simulink model "Thruster_Example_rw"  (R2024b)
settings: Solver=ode4  StartTime=0.0  StopTime=2000  FixedStep=0.01  RelTol=1e-3
undefined symbols (not defined in the file): Cube_L, dt, F_vec, Iws, M_rw, m_tot, norm_Ib, Omega1_init, Omega2_init, Omega3_init, Omega4_init, qb0, rad2rpm, RCS_F, RCS_F_vec, RCS_Pos, RCS_pos, RCS_PWM_Freq, RCS_Sampling_time, RCS_THR_vec, REL_TS_POS_I_0, REL_TS_VEL_I_0, RW_As, RW_Max_Speed, RW_Omegad_max, sat, SC_Ib, SC_state0, SS_Total_Mass, TC_Kepler, THR_dt, THR_Force, THR_freq, THR_Pos, TS_Ib, TS_qb0, TS_state0, TS_wb0, wb0, X, Y, Z
libraries: sm_lib x348, nesl_utility x236, simulink_extras x115, sharedtransform x64, aerolibutil x38, simulink x28, sharedutil x13
(part 8 of 16)

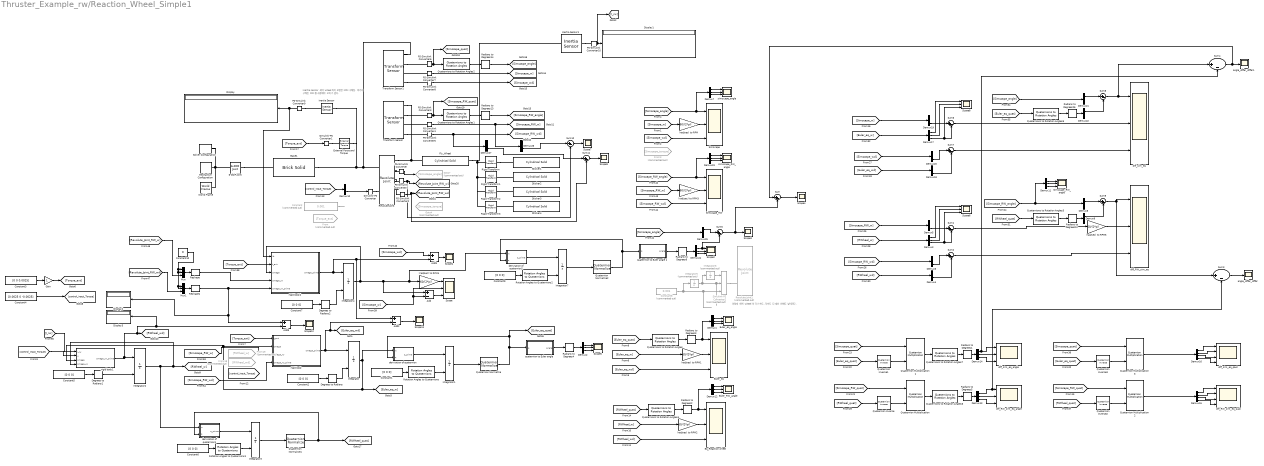
== system Thruster_Example_rw/Reaction_Wheel_Simple1 ==
  note: inertia sensor 써야 wheel까지 포함한 MOI 구해짐.
      | 여기서 구해진 MOI를 사용해야 오차가 없다.
  note: 이렇게 하면, wheel의 각가속도, 각속도 다 계산 안해도 넣어진다.
  (rad/sec) to RPM{,1..5} (6 alike) : Gain  Gain=60/(2*pi)
  6-DOF Joint : sm_lib/Joints/6-DOF Joint  JointMode=Normal  CompositeWrenchDir=FollowerOnBase  CompositeWrenchFrame=BaseFrame  SenseConstraintForce=off  SenseConstraintTorque=off  SenseTotalForce=off  SenseTotalTorque=off  PxPositionTargetSpecify=off  PxPositionTargetPriority=High  PxPositionTargetValue=0  PxPositionTargetValueUnits=m  PxVelocityTargetSpecify=off  PxVelocityTargetPriority=High  PxVelocityTargetValue=0  PxVelocityTargetValueUnits=m/s  PxEquilibriumPosition=0  PxEquilibriumPositionUnits=m  PxSpringStiffness=0  PxSpringStiffnessUnits=N/m  PxDampingCoefficient=0  PxDampingCoefficientUnits=N/(m/s)  PxLowerLimitSpecify=off  PxLowerLimitBound=-1  PxLowerLimitBoundUnits=m  PxLowerLimitStiffness=1e6  PxLowerLimitStiffnessUnits=N/m  PxLowerLimitDamping=1e3  PxLowerLimitDampingUnits=N/(m/s)  PxLowerLimitTransitionRegionWidth=1e-4  PxLowerLimitTransitionRegionWidthUnits=m  PxUpperLimitSpecify=off  PxUpperLimitBound=1  PxUpperLimitBoundUnits=m  PxUpperLimitStiffness=1e6  PxUpperLimitStiffnessUnits=N/m  PxUpperLimitDamping=1e3  PxUpperLimitDampingUnits=N/(m/s)  PxUpperLimitTransitionRegionWidth=1e-4  PxUpperLimitTransitionRegionWidthUnits=m  PxTorqueActuationMode=NoTorque  PxMotionActuationMode=ComputedMotion  PxSensePosition=off  PxSenseVelocity=off  PxSenseAcceleration=off  PxSenseTorqueForce=off  PxSenseLowerLimitTorqueForce=off  PxSenseUpperLimitTorqueForce=off  PyPositionTargetSpecify=off  PyPositionTargetPriority=High  PyPositionTargetValue=0  PyPositionTargetValueUnits=m  PyVelocityTargetSpecify=off  PyVelocityTargetPriority=High  PyVelocityTargetValue=0  PyVelocityTargetValueUnits=m/s  PyEquilibriumPosition=0  PyEquilibriumPositionUnits=m  PySpringStiffness=0  PySpringStiffnessUnits=N/m  PyDampingCoefficient=0  PyDampingCoefficientUnits=N/(m/s)  PyLowerLimitSpecify=off  PyLowerLimitBound=-1  PyLowerLimitBoundUnits=m  PyLowerLimitStiffness=1e6  PyLowerLimitStiffnessUnits=N/m  PyLowerLimitDamping=1e3  PyLowerLimitDampingUnits=N/(m/s)  PyLowerLimitTransitionRegionWidth=1e-4  PyLowerLimitTransitionRegionWidthUnits=m  PyUpperLimitSpecify=off  PyUpperLimitBound=1  PyUpperLimitBoundUnits=m  PyUpperLimitStiffness=1e6  PyUpperLimitStiffnessUnits=N/m  PyUpperLimitDamping=1e3  PyUpperLimitDampingUnits=N/(m/s)  PyUpperLimitTransitionRegionWidth=1e-4  PyUpperLimitTransitionRegionWidthUnits=m  PyTorqueActuationMode=NoTorque  PyMotionActuationMode=ComputedMotion  PySensePosition=off  PySenseVelocity=off  PySenseAcceleration=off  PySenseTorqueForce=off  PySenseLowerLimitTorqueForce=off  PySenseUpperLimitTorqueForce=off  PzPositionTargetSpecify=off  PzPositionTargetPriority=High  PzPositionTargetValue=0  PzPositionTargetValueUnits=m  PzVelocityTargetSpecify=off  PzVelocityTargetPriority=High  PzVelocityTargetValue=0  PzVelocityTargetValueUnits=m/s  PzEquilibriumPosition=0  PzEquilibriumPositionUnits=m  PzSpringStiffness=0  PzSpringStiffnessUnits=N/m  PzDampingCoefficient=0  PzDampingCoefficientUnits=N/(m/s)  PzLowerLimitSpecify=off  PzLowerLimitBound=-1  PzLowerLimitBoundUnits=m  PzLowerLimitStiffness=1e6  PzLowerLimitStiffnessUnits=N/m  PzLowerLimitDamping=1e3  PzLowerLimitDampingUnits=N/(m/s)  PzLowerLimitTransitionRegionWidth=1e-4  PzLowerLimitTransitionRegionWidthUnits=m  PzUpperLimitSpecify=off  PzUpperLimitBound=1  PzUpperLimitBoundUnits=m  PzUpperLimitStiffness=1e6  PzUpperLimitStiffnessUnits=N/m  PzUpperLimitDamping=1e3  PzUpperLimitDampingUnits=N/(m/s)  PzUpperLimitTransitionRegionWidth=1e-4  PzUpperLimitTransitionRegionWidthUnits=m  PzTorqueActuationMode=NoTorque  PzMotionActuationMode=ComputedMotion  PzSensePosition=off  PzSenseVelocity=off  PzSenseAcceleration=off  PzSenseTorqueForce=off  PzSenseLowerLimitTorqueForce=off  PzSenseUpperLimitTorqueForce=off  SphPositionTargetSpecify=off  SphPositionTargetPriority=High  SphPositionTargetRotationMethod=None  SphPositionTargetFollAlignAxisA=+X  SphPositionTargetBaseAlignAxisA=+Y  SphPositionTargetFollAlignAxisB=+Y  SphPositionTargetBaseAlignAxisB=+Z  SphPositionTargetRotationStandardAxis=+Z  SphPositionTargetRotationAngle=0.0  SphPositionTargetRotationAngleUnits=deg  SphPositionTargetRotationArbitraryAxis=[0 0 1]  SphPositionTargetRotationSequenceAxes=FollowerAxes  SphPositionTargetRotationSequence=XYX  SphPositionTargetRotationSequenceAngles=[0 0 0]  SphPositionTargetRotationSequenceAnglesUnits=deg  SphPositionTargetRotationMatrix=[1 0 0; 0 1 0; 0 0 1]  SphPositionTargetQuaternion=[1 0 0 0]  SphVelocityTargetSpecify=off  SphVelocityTargetPriority=High  SphVelocityTargetValue=[0 0 0]  SphVelocityTargetValueUnits=deg/s  SphVelocityTargetInFollowerFrame=on  SphEqPosRotationMethod=None  SphEqPosFollAlignAxisA=+X  SphEqPosBaseAlignAxisA=+Y  SphEqPosFollAlignAxisB=+Y  SphEqPosBaseAlignAxisB=+Z  SphEqPosRotationStandardAxis=+Z  SphEqPosRotationAngle=0.0  SphEqPosRotationAngleUnits=deg  SphEqPosRotationArbitraryAxis=[0 0 1]  SphEqPosRotationSequenceAxes=FollowerAxes  SphEqPosRotationSequence=XYX  SphEqPosRotationSequenceAngles=[0 0 0]  SphEqPosRotationSequenceAnglesUnits=deg  SphEqPosRotationMatrix=[1 0 0; 0 1 0; 0 0 1]  SphEqPosQuaternion=[1 0 0 0]  SphSpringStiffness=0  SphSpringStiffnessUnits=N*m/deg  SphDampingCoefficient=0  SphDampingCoefficientUnits=N*m/(deg/s)  SphLowerLimitSpecify=off  SphLowerLimitBound=15  SphLowerLimitBoundUnits=deg  SphLowerLimitStiffness=1e4  SphLowerLimitStiffnessUnits=N*m/deg  SphLowerLimitDamping=10  SphLowerLimitDampingUnits=N*m/(deg/s)  SphLowerLimitTransitionRegionWidth=0.1  SphLowerLimitTransitionRegionWidthUnits=deg  SphUpperLimitSpecify=off  SphUpperLimitBound=45  SphUpperLimitBoundUnits=deg  SphUpperLimitStiffness=1e4  SphUpperLimitStiffnessUnits=N*m/deg  SphUpperLimitDamping=10  SphUpperLimitDampingUnits=N*m/(deg/s)  SphUpperLimitTransitionRegionWidth=0.1  SphUpperLimitTransitionRegionWidthUnits=deg  SphTorqueActuationMode=NoTorque  SphActuateTorqueX=off  SphActuateTorqueY=off  SphActuateTorqueZ=on  SphActuateTorque=off  SphActuationFrame=BaseFrame  SphSensePosition=off  SphSenseVelocityX=off  SphSenseVelocityY=off  SphSenseVelocityZ=off  SphSenseVelocity=off  SphSenseAccelerationX=off  SphSenseAccelerationY=off  SphSenseAccelerationZ=off  SphSenseAcceleration=off  SphSenseLowerLimitTorqueMag=off  SphSenseUpperLimitTorqueMag=off  SphSensingFrame=BaseFrame
  Add{,1..3} (4 alike) : Sum  Inputs=+-
  Base1 : sm_lib/Body Elements/Brick Solid  BrickDimensions=[0.3 0.3 0.3]  BrickDimensionsUnits=m  ExportEntireGeometry=off  InertiaType=CalculateFromGeometry  BasedOnType=Mass  Density=1000  DensityUnits=kg/m^3  Mass=10  MassUnits=kg  CenterOfMass=[0 0 0]  CenterOfMassUnits=m  MomentsOfInertia=[1 1 1]  MomentsOfInertiaUnits=kg*m^2  ProductsOfInertia=[0 0 0]  ProductsOfInertiaUnits=kg*m^2  GraphicType=FromGeometry  MarkerShape=Sphere  MarkerSize=10  GraphicVisPropType=SimpleVisualProperties  GraphicDiffuseColor=[0.0 0.8 0.8]  GraphicOpacity=0.2  GraphicSpecularColor=[0.5 0.5 0.5 1.0]  GraphicAmbientColor=[0.15 0.15 0.15 1.0]  GraphicEmissiveColor=[0.0 0.0 0.0 1.0]  GraphicShininess=75  DoExposeReferenceFrame=on  SerializedFrames=<Frames><Frame><Id>Frame1</Id><Value><Name>CM_F</Name><Origin><Source>CenterOfMassFrame</Source><FeatureName></FeatureName></Origin><PrimaryAxis><DefinedDirection>+Z</DefinedDirection><Source>ReferenceFrame</Source><SourceDirection>+Z</SourceDirection><FeatureName></FeatureName></PrimaryAxis><SecondaryAxis><DefinedDirection>+X</DefinedDirection><Source>ReferenceFrame</Source><SourceDirection>+X</SourceDirection><FeatureName></FeatureName></SecondaryAxis></Value></Frame></Frames>
  Constant : Constant  Commented=on  Value=0.001
  Constant{1..2,5..7,9} (6 alike) : Constant  Value=[0 0 0]
  Constant10 : Constant  Value=0
  Constant3 : Constant  Value=[0 0 0.0025]
  Constant4 : Constant  Value=[0.0025 0 -0.0025]
  Constant8 : Constant  Commented=on  Value=0.001
  Degrees to Radians : simulink_extras/Transformations/Degrees to Radians
  Degrees to Radians1 : simulink_extras/Transformations/Degrees to Radians
  Degrees to Radians2 : simulink_extras/Transformations/Degrees to Radians
  Demux{1..14,17..27} (25 alike) : Demux  Outputs=3
  Demux15 : Demux
  Demux16 : Demux
  Display{,1..3} (4 alike) : Display
  Eq_Reaction wheel : Scope  NumInputPorts=3
  Euler_RW_angle : Scope  NumInputPorts=3
  Euler_eq : Scope  NumInputPorts=3
  Euler_eq_angle : Scope  NumInputPorts=3
  External Force and Torque : sm_lib/Forces and Torques/External Force and Torque  EnableForceX=off  EnableForceY=off  EnableForceZ=off  EnableForce=off  ForceResolutionFrame=World  EnableTorqueX=off  EnableTorqueY=off  EnableTorqueZ=off  EnableTorque=on  TorqueResolutionFrame=World
  Fly_Wheel : sm_lib/Body Elements/Cylindrical Solid  CylinderRadius=0.015  CylinderRadiusUnits=m  CylinderLength=0.01  CylinderLengthUnits=m  ExportEntireGeometry=off  InertiaType=CalculateFromGeometry  BasedOnType=Mass  Density=1000  DensityUnits=kg/m^3  Mass=0.01  MassUnits=kg  CenterOfMass=[0 0 0]  CenterOfMassUnits=m  MomentsOfInertia=[1 1 1]  MomentsOfInertiaUnits=kg*m^2  ProductsOfInertia=[0 0 0]  ProductsOfInertiaUnits=kg*m^2  GraphicType=FromGeometry  MarkerShape=Sphere  MarkerSize=10  GraphicVisPropType=SimpleVisualProperties  GraphicDiffuseColor=[0.0 0.0 1.0]  GraphicOpacity=1.0  GraphicSpecularColor=[0.5 0.5 0.5 1.0]  GraphicAmbientColor=[0.15 0.15 0.15 1.0]  GraphicEmissiveColor=[0.0 0.0 0.0 1.0]  GraphicShininess=75  DoExposeReferenceFrame=on  SerializedFrames=<Frames><Frame><Id>Frame1</Id><Value><Name>Sticker_F</Name><Origin><Source>GeometricFeature</Source><FeatureName>top surface</FeatureName></Origin><PrimaryAxis><DefinedDirection>+Z</DefinedDirection><Source>ReferenceFrame</Source><SourceDirection>+Z</SourceDirection><FeatureName></FeatureName></PrimaryAxis><SecondaryAxis><DefinedDirection>+X</DefinedDirection><Source>ReferenceFrame</Source><SourceDirection>+X</SourceDirection><FeatureName></FeatureName></SecondaryAxis></Value></Frame></Frames>
  From : From  Commented=on  GotoTag=Torque_ext
  From18 : From  Commented=on  GotoTag=RWheel_wd
  From19 : From  Commented=on  GotoTag=RWheel_w
  From3 : From  Commented=on  GotoTag=Simscape_torque
  Gain : Gain
  Goto4 : Goto  Commented=on  GotoTag=Simscape_torque
  Goto7 : Goto  Commented=on  GotoTag=Simscape_angle
  Inertia Sensor : sm_lib/Body Elements/Inertia Sensor  SensorExtent=Mechanism  SpanWeldJoints=off  ExcludeGroundedBodies=off  MeasurementFrame=Attached  SenseMass=off  SenseCenterOfMass=off  SenseInertiaMatrix=on  SenseCenteredInertiaMatrix=off  SensePrincipalInertiaMatrix=off  SenseRotationMatrix=off  GraphicType=PrincipalInertiaFrame  PrincipalInertiaFrameSize=20  GraphicVisPropType=SimpleVisualProperties  GraphicDiffuseColor=[0.5 0.5 0.5]  GraphicOpacity=1.0  GraphicSpecularColor=[0.5 0.5 0.5 1.0]  GraphicAmbientColor=[0.15 0.15 0.15 1.0]  GraphicEmissiveColor=[0.0 0.0 0.0 1.0]  GraphicShininess=75
  Inertia Sensor1 : sm_lib/Body Elements/Inertia Sensor  SensorExtent=BodyGroup  SpanWeldJoints=off  ExcludeGroundedBodies=off  MeasurementFrame=Attached  SenseMass=off  SenseCenterOfMass=off  SenseInertiaMatrix=on  SenseCenteredInertiaMatrix=off  SensePrincipalInertiaMatrix=off  SenseRotationMatrix=off  GraphicType=PrincipalInertiaFrame  PrincipalInertiaFrameSize=20  GraphicVisPropType=SimpleVisualProperties  GraphicDiffuseColor=[0.5 0.5 0.5]  GraphicOpacity=1.0  GraphicSpecularColor=[0.5 0.5 0.5 1.0]  GraphicAmbientColor=[0.15 0.15 0.15 1.0]  GraphicEmissiveColor=[0.0 0.0 0.0 1.0]  GraphicShininess=75
  Integrator{,1..4,7} (6 alike) : Integrator  InitialConditionSource=external
  Integrator5 : Integrator  Commented=on
  Integrator6 : Integrator  Commented=on
  Mechanism Configuration : sm_lib/Utilities/Mechanism Configuration  UniformGravity=None  GravityVector=[0 0 -9.80665]  GravityVectorUnits=m/s^2  LinearizationDelta=0.001  JointModeTransitionNonlinearIterations=2
  Mux : Mux  Inputs=3
  Mux1 : Mux  Inputs=3
  PS-Simulink Converter{,1..10} (11 alike) : nesl_utility/PS-Simulink Converter  PhysicalDomain=network_engine_domain  SubClassName=ps_output  LeftPortType=input  RightPortType=output  PseudoPeriodic=off  Frequencies=[]  VectorFormat=inherit  Unit=inherit  AffineConversion=off
  Quaternion Inverse{,1..3} (4 alike) : aerolibutil/Quaternion Inverse
  Quaternion Multiplication{,1..3} (4 alike) : aerolibutil/Quaternion Multiplication
  Quaternion Normalize : sharedutil/Quaternion Normalize  aMode=aMode
  Quaternion Normalize1 : sharedutil/Quaternion Normalize  aMode=aMode
  Quaternion Normalize2 : sharedutil/Quaternion Normalize  aMode=aMode
  Quaternions to Rotation Angles{,1..7} (8 alike) : sharedtransform/Quaternions to Rotation Angles  rotationOrder=ZYX  aMode=aMode
  Radians to Degrees{1..6,12..14,26} (10 alike) : simulink_extras/Transformations/Radians to Degrees
  Reshape : Reshape  OutputDimensionality=Column vector (2-D)
  Reshape1 : Reshape  OutputDimensionality=Column vector (2-D)
  Revolute Joint : sm_lib/Joints/Revolute Joint  JointMode=Normal  CompositeWrenchDir=FollowerOnBase  CompositeWrenchFrame=BaseFrame  SenseConstraintForce=off  SenseConstraintTorque=off  SenseTotalForce=off  SenseTotalTorque=off  PositionTargetSpecify=off  PositionTargetPriority=High  PositionTargetValue=0  PositionTargetValueUnits=deg  VelocityTargetSpecify=off  VelocityTargetPriority=High  VelocityTargetValue=0  VelocityTargetValueUnits=deg/s  EquilibriumPosition=0  EquilibriumPositionUnits=deg  SpringStiffness=0  SpringStiffnessUnits=N*m/deg  DampingCoefficient=0  DampingCoefficientUnits=N*m/(deg/s)  LowerLimitSpecify=off  LowerLimitBound=-90  LowerLimitBoundUnits=deg  LowerLimitStiffness=1e4  LowerLimitStiffnessUnits=N*m/deg  LowerLimitDamping=10  LowerLimitDampingUnits=N*m/(deg/s)  LowerLimitTransitionRegionWidth=0.1  LowerLimitTransitionRegionWidthUnits=deg  UpperLimitSpecify=off  UpperLimitBound=90  UpperLimitBoundUnits=deg  UpperLimitStiffness=1e4  UpperLimitStiffnessUnits=N*m/deg  UpperLimitDamping=10  UpperLimitDampingUnits=N*m/(deg/s)  UpperLimitTransitionRegionWidth=0.1  UpperLimitTransitionRegionWidthUnits=deg  TorqueActuationMode=InputTorque  MotionActuationMode=ComputedMotion  SensePosition=on  SenseVelocity=on  SenseAcceleration=on  SenseTorqueForce=on  SenseLowerLimitTorqueForce=off  SenseUpperLimitTorqueForce=off
  Revolute Joint1 : sm_lib/Joints/Revolute Joint  Commented=on  JointMode=Normal  CompositeWrenchDir=FollowerOnBase  CompositeWrenchFrame=BaseFrame  SenseConstraintForce=off  SenseConstraintTorque=off  SenseTotalForce=off  SenseTotalTorque=off  PositionTargetSpecify=off  PositionTargetPriority=High  PositionTargetValue=0  PositionTargetValueUnits=deg  VelocityTargetSpecify=off  VelocityTargetPriority=High  VelocityTargetValue=0  VelocityTargetValueUnits=deg/s  EquilibriumPosition=0  EquilibriumPositionUnits=deg  SpringStiffness=0  SpringStiffnessUnits=N*m/deg  DampingCoefficient=0  DampingCoefficientUnits=N*m/(deg/s)  LowerLimitSpecify=off  LowerLimitBound=-90  LowerLimitBoundUnits=deg  LowerLimitStiffness=1e4  LowerLimitStiffnessUnits=N*m/deg  LowerLimitDamping=10  LowerLimitDampingUnits=N*m/(deg/s)  LowerLimitTransitionRegionWidth=0.1  LowerLimitTransitionRegionWidthUnits=deg  UpperLimitSpecify=off  UpperLimitBound=90  UpperLimitBoundUnits=deg  UpperLimitStiffness=1e4  UpperLimitStiffnessUnits=N*m/deg  UpperLimitDamping=10  UpperLimitDampingUnits=N*m/(deg/s)  UpperLimitTransitionRegionWidth=0.1  UpperLimitTransitionRegionWidthUnits=deg  TorqueActuationMode=ComputedTorque  MotionActuationMode=InputMotion  SensePosition=on  SenseVelocity=on  SenseAcceleration=on  SenseTorqueForce=on  SenseLowerLimitTorqueForce=off  SenseUpperLimitTorqueForce=off
  Rigid Transform : sm_lib/Frames and Transforms/Rigid Transform  RotationMethod=None  FollAlignAxisA=+X  BaseAlignAxisA=+Y  FollAlignAxisB=+Y  BaseAlignAxisB=+Z  RotationStandardAxis=+Z  RotationAngle=0.0  RotationAngleUnits=deg  RotationArbitraryAxis=[0 0 1]  RotationSequenceAxes=FollowerAxes  RotationSequence=XYX  RotationSequenceAngles=[0 0 0]  RotationSequenceAnglesUnits=deg  RotationMatrix=[1 0 0; 0 1 0; 0 0 1]  Quaternion=[1 0 0 0]  TranslationMethod=Cartesian  TranslationCartesianOffset=[0.01 0 0]  TranslationCartesianOffsetUnits=m  TranslationStandardAxis=+Z  TranslationStandardOffset=0  TranslationStandardOffsetUnits=m  TranslationROffset=0  TranslationROffsetUnits=m  TranslationThetaOffset=0  TranslationThetaOffsetUnits=deg  TranslationZOffset=0  TranslationZOffsetUnits=m
  Rigid Transform1 : sm_lib/Frames and Transforms/Rigid Transform  RotationMethod=None  FollAlignAxisA=+X  BaseAlignAxisA=+Y  FollAlignAxisB=+Y  BaseAlignAxisB=+Z  RotationStandardAxis=+Z  RotationAngle=0.0  RotationAngleUnits=deg  RotationArbitraryAxis=[0 0 1]  RotationSequenceAxes=FollowerAxes  RotationSequence=XYX  RotationSequenceAngles=[0 0 0]  RotationSequenceAnglesUnits=deg  RotationMatrix=[1 0 0; 0 1 0; 0 0 1]  Quaternion=[1 0 0 0]  TranslationMethod=Cartesian  TranslationCartesianOffset=[-0.01 0 0]  TranslationCartesianOffsetUnits=m  TranslationStandardAxis=+Z  TranslationStandardOffset=0  TranslationStandardOffsetUnits=m  TranslationROffset=0  TranslationROffsetUnits=m  TranslationThetaOffset=0  TranslationThetaOffsetUnits=deg  TranslationZOffset=0  TranslationZOffsetUnits=m
  Rigid Transform2 : sm_lib/Frames and Transforms/Rigid Transform  RotationMethod=None  FollAlignAxisA=+X  BaseAlignAxisA=+Y  FollAlignAxisB=+Y  BaseAlignAxisB=+Z  RotationStandardAxis=+Z  RotationAngle=0.0  RotationAngleUnits=deg  RotationArbitraryAxis=[0 0 1]  RotationSequenceAxes=FollowerAxes  RotationSequence=XYX  RotationSequenceAngles=[0 0 0]  RotationSequenceAnglesUnits=deg  RotationMatrix=[1 0 0; 0 1 0; 0 0 1]  Quaternion=[1 0 0 0]  TranslationMethod=Cartesian  TranslationCartesianOffset=[0 0.01 0]  TranslationCartesianOffsetUnits=m  TranslationStandardAxis=+Z  TranslationStandardOffset=0  TranslationStandardOffsetUnits=m  TranslationROffset=0  TranslationROffsetUnits=m  TranslationThetaOffset=0  TranslationThetaOffsetUnits=deg  TranslationZOffset=0  TranslationZOffsetUnits=m
  Rigid Transform3 : sm_lib/Frames and Transforms/Rigid Transform  RotationMethod=None  FollAlignAxisA=+X  BaseAlignAxisA=+Y  FollAlignAxisB=+Y  BaseAlignAxisB=+Z  RotationStandardAxis=+Z  RotationAngle=0.0  RotationAngleUnits=deg  RotationArbitraryAxis=[0 0 1]  RotationSequenceAxes=FollowerAxes  RotationSequence=XYX  RotationSequenceAngles=[0 0 0]  RotationSequenceAnglesUnits=deg  RotationMatrix=[1 0 0; 0 1 0; 0 0 1]  Quaternion=[1 0 0 0]  TranslationMethod=Cartesian  TranslationCartesianOffset=[0 -0.01 0]  TranslationCartesianOffsetUnits=m  TranslationStandardAxis=+Z  TranslationStandardOffset=0  TranslationStandardOffsetUnits=m  TranslationROffset=0  TranslationROffsetUnits=m  TranslationThetaOffset=0  TranslationThetaOffsetUnits=deg  TranslationZOffset=0  TranslationZOffsetUnits=m
  Rotation Angles to Quaternions : sharedtransform/Rotation Angles to Quaternions  rotationOrder=ZYX  aMode=aMode
  Rotation Angles to Quaternions1 : sharedtransform/Rotation Angles to Quaternions  rotationOrder=ZYX  aMode=aMode
  Rotation Angles to Quaternions2 : sharedtransform/Rotation Angles to Quaternions  rotationOrder=ZYX  aMode=aMode
  Scope{,2,5..6,8} (5 alike) : Scope  NumInputPorts=3
  Scope{1,3..4,7,9,11..12} (7 alike) : Scope
  Simscape : Scope  NumInputPorts=3
  Simscape_RW : Scope  NumInputPorts=3
  Simscape_RW_angle : Scope  NumInputPorts=3
  Simulink-PS Converter : nesl_utility/Simulink-PS Converter  PhysicalDomain=network_engine_domain  SubClassName=ps_input  LeftPortType=input  RightPortType=output  PseudoPeriodic=off  Frequencies=[]  NoiseDistribution=none  NoiseParameters=[]  Unit=1  AffineConversion=off  FilteringAndDerivatives=provide  SimscapeFilterOrder=1  InputFilterTimeConstant=0.001  UdotUserProvided=0
  Simulink-PS Converter1 : nesl_utility/Simulink-PS Converter  PhysicalDomain=network_engine_domain  SubClassName=ps_input  LeftPortType=input  RightPortType=output  PseudoPeriodic=off  Frequencies=[]  NoiseDistribution=none  NoiseParameters=[]  Unit=1  AffineConversion=off  FilteringAndDerivatives=provide  SimscapeFilterOrder=1  InputFilterTimeConstant=0.001  UdotUserProvided=0
  Simulink-PS Converter2 : nesl_utility/Simulink-PS Converter  Commented=on  PhysicalDomain=network_engine_domain  SubClassName=ps_input  LeftPortType=input  RightPortType=output  PseudoPeriodic=off  Frequencies=[]  NoiseDistribution=none  NoiseParameters=[]  Unit=1  AffineConversion=off  FilteringAndDerivatives=provide  SimscapeFilterOrder=1  InputFilterTimeConstant=0.001  UdotUserProvided=2
  Solver Configuration : nesl_utility/Solver Configuration  PhysicalDomain=network_engine_domain  SubClassName=solver  LeftPortType=input  RightPortType=generic  Tones=[]  Harmonics=[]  SimulateNoise=off  Profile=off  UseLocalSampling=off  EnableSwitchedLinearOptims=on  FrequencyDomain=off  UseCCode=off  RelTol=0.001  AbsTol=0.001  MinStep=1e-09  ToWorkspace=off  RevertToSquareIcSolve=off  NumHomotopyIterations=100  PhasorMode=off  PhasorModeNumHarmonics=1  ConsistencySolver=NEWTON_XTOL_AFTER_FTOL  IndexReductionMethod=DerivativeReplacement  DoDC=off  ResidualTolerance=1e-09  ConsistencyTolSource=GLOBAL  ConsistencyAbsTol=0.001  ConsistencyRelTol=0.001  ConsistencyTolFactor=0.001  UseLocalSolver=off  LocalSolverChoice=NE_BACKWARD_EULER_ADVANCER  ResolveIndetEquations=on  FunctionEvalNumThread=1  LocalSolverSampleTime=0.001  DoFixedCost=off  MaxNonlinIter=3  MaxModeIter=2  ComputeImpulses=off  ImpulseIterations=2  LinearAlgebra=auto  LinearAlgebraNumThread=0  EquationFormulation=NE_TIME_EF  DelaysMemoryBudget=1024  AutomaticFiltering=on  FilteringTimeConstant=0.001  PartitionStorageMethod=AS_NEEDED  PartitionMemoryBudget=1024  PartitionMethod=ROBUST  MultibodyUseLocalSolver=off  MultibodyLocalSolverChoice=ODE1  MultibodyLocalSolverSampleTime=0.001
  Sticker{1..4} (4 alike) : sm_lib/Body Elements/Cylindrical Solid  CylinderRadius=0.003  CylinderRadiusUnits=m  CylinderLength=0.00001  CylinderLengthUnits=m  ExportEntireGeometry=off  InertiaType=CalculateFromGeometry  BasedOnType=Mass  Density=1000  DensityUnits=kg/m^3  Mass=0.000000000000000000000000000000000000000000000000000000000000000001  MassUnits=kg  CenterOfMass=[0 0 0]  CenterOfMassUnits=m  MomentsOfInertia=[1 1 1]  MomentsOfInertiaUnits=kg*m^2  ProductsOfInertia=[0 0 0]  ProductsOfInertiaUnits=kg*m^2  GraphicType=FromGeometry  MarkerShape=Sphere  MarkerSize=10  GraphicVisPropType=SimpleVisualProperties  GraphicDiffuseColor=[1.0 1.0 0.2]  GraphicOpacity=1.0  GraphicSpecularColor=[0.5 0.5 0.5 1.0]  GraphicAmbientColor=[0.15 0.15 0.15 1.0]  GraphicEmissiveColor=[0.0 0.0 0.0 1.0]  GraphicShininess=75  DoExposeReferenceFrame=on  SerializedFrames=<Frames><Frame><Id>Frame1</Id><Value><Name>Sticker_F</Name><Origin><Source>GeometricFeature</Source><FeatureName>bottom surface</FeatureName></Origin><PrimaryAxis><DefinedDirection>+Z</DefinedDirection><Source>ReferenceFrame</Source><SourceDirection>+Z</SourceDirection><FeatureName></FeatureName></PrimaryAxis><SecondaryAxis><DefinedDirection>+X</DefinedDirection><Source>ReferenceFrame</Source><SourceDirection>+X</SourceDirection><FeatureName></FeatureName></SecondaryAxis></Value></Frame></Frames>
  Sum{,1..11} (12 alike) : Sum  Inputs=|+-
  Transform Sensor : sm_lib/Frames and Transforms/Transform Sensor  MeasurementFrame=World  RotationSequence=ZYX  SenseAngle=off  SenseAxis=off  SenseQ=on  SenseR=off  SenseRotationSequence=off  SenseOmegaX=off  SenseOmegaY=off  SenseOmegaZ=off  SenseOmega=on  SenseQDot=off  SenseRDot=off  SenseRotationSequenceDot=off  SenseAlphaX=off  SenseAlphaY=off  SenseAlphaZ=off  SenseAlpha=on  SenseQDDot=off  SenseRDDot=off  SenseX=off  SenseY=off  SenseZ=off  SenseXYZ=off  SenseRad=off  SenseAzim=off  SenseDist=off  SenseInc=off  SenseXDot=off  SenseYDot=off  SenseZDot=off  SenseXYZDot=off  SenseRadDot=off  SenseAzimDot=off  SenseDistDot=off  SenseIncDot=off  SenseXDDot=off  SenseYDDot=off  SenseZDDot=off  SenseXYZDDot=off  SenseRadDDot=off  SenseAzimDDot=off  SenseDistDDot=off  SenseIncDDot=off
  Transform Sensor1 : sm_lib/Frames and Transforms/Transform Sensor  MeasurementFrame=World  RotationSequence=ZYX  SenseAngle=off  SenseAxis=off  SenseQ=on  SenseR=off  SenseRotationSequence=off  SenseOmegaX=off  SenseOmegaY=off  SenseOmegaZ=off  SenseOmega=on  SenseQDot=off  SenseRDot=off  SenseRotationSequenceDot=off  SenseAlphaX=off  SenseAlphaY=off  SenseAlphaZ=off  SenseAlpha=on  SenseQDDot=off  SenseRDDot=off  SenseX=off  SenseY=off  SenseZ=off  SenseXYZ=off  SenseRad=off  SenseAzim=off  SenseDist=off  SenseInc=off  SenseXDot=off  SenseYDot=off  SenseZDot=off  SenseXYZDot=off  SenseRadDot=off  SenseAzimDot=off  SenseDistDot=off  SenseIncDot=off  SenseXDDot=off  SenseYDDot=off  SenseZDDot=off  SenseXYZDDot=off  SenseRadDDot=off  SenseAzimDDot=off  SenseDistDDot=off  SenseIncDDot=off
  World Frame : sm_lib/Frames and Transforms/World Frame
  angle_differ_differ : Scope
  angle_differ_differ1 : Scope
  deriviation of quaternion : MATLAB Function  TreatAsAtomicUnit=on
  deriviation of quaternion1 : MATLAB Function  TreatAsAtomicUnit=on
  deriviation of quaternion2 : MATLAB Function  TreatAsAtomicUnit=on
  diff_RW_sim_eq : Scope  NumInputPorts=3
  diff_RW_sim_eq_angle : Scope  NumInputPorts=3
  diff_RW_sim_eq_quat : Scope  NumInputPorts=4
  diff_sim_eq : Scope  NumInputPorts=3
  diff_sim_eq_angle : Scope  NumInputPorts=3
  diff_sim_eq_qaut : Scope  NumInputPorts=4
  "quaternion to Euler angle " : MATLAB Function  TreatAsAtomicUnit=on
  quaternion to Euler angle 1 : MATLAB Function  TreatAsAtomicUnit=on
  rigid body : MATLAB Function  TreatAsAtomicUnit=on
  rigid body1 : MATLAB Function  TreatAsAtomicUnit=on
  rigid body2 : MATLAB Function  TreatAsAtomicUnit=on
  simscape_RW_angle : Scope  NumInputPorts=3
  simscape_angle : Scope  NumInputPorts=3
  wires:
  "quaternion to Euler angle "/1(angle) -> Radians to Degrees4/1
  Demux2/1 -> Scope5/1
  Quaternion Normalize/1 -> "quaternion to Euler angle "/1(q), [Euler_eq_quat], deriviation of quaternion/2(q)
  Constant1/1 -> Rotation Angles to Quaternions/1
  Rotation Angles to Quaternions/1 -> Integrator1/2
  rigid body/1(omega_prime) -> Integrator/1, Add2/2, [Euler_eq_wd]
  Radians to Degrees4/1 -> Demux2/1
  Demux2/3 -> Scope5/3
  Integrator1/1 -> Quaternion Normalize/1
  Demux2/2 -> Scope5/2
  [Torque_ext] -> rigid body/1(t_ext)
  deriviation of quaternion/1(q_prime) -> Integrator1/1
  Integrator/1 -> rigid body1/3(omega), rigid body/2(omega), [Euler_eq_w], deriviation of quaternion/1(w)
  Degrees to Radians/1 -> Integrator/2
  Constant2/1 -> Degrees to Radians/1
  PS-Simulink Converter/1 -> Goto7/1
  PS-Simulink Converter2/1 -> [Revolute_Joint_RW_wd], Sum11/2
  PS-Simulink Converter1/1 -> [Revolute_Joint_RW_w], Sum10/2
  [Simscape_wd] -> Simscape/3
  [Simscape_w] -> (rad/sec) to RPM/1
  [Simscape_angle] -> Demux7/1, Simscape/1
  [Euler_eq_w] -> (rad/sec) to RPM1/1
  [Euler_eq_wd] -> Euler_eq/3
  Demux1/1 -> Euler_eq_angle/1
  Demux1/2 -> Euler_eq_angle/2
  Demux1/3 -> Euler_eq_angle/3
  [Euler_eq_quat] -> Quaternions to Rotation Angles/1
  Quaternions to Rotation Angles/1 -> Radians to Degrees3/1
  Radians to Degrees3/1 -> Demux1/1, Euler_eq/1
  Constant4/1 -> [control_input_Torque]
  [control_input_Torque] -> rigid body1/2(u)
  Degrees to Radians1/1 -> Integrator2/2
  Constant5/1 -> Degrees to Radians1/1
  rigid body1/1(omega_rw_prime) -> Display3/1, Add3/2, [RWheel_wd], Integrator2/1
  Integrator2/1 -> deriviation of quaternion1/1(w), rigid body1/4(omega_rw), [RWheel_w]
  [RWheel_wd] -> Eq_Reaction wheel/3
  [RWheel_w] -> (rad/sec) to RPM2/1
  PS-Simulink Converter3/1 -> [Simscape_RW_quat], Quaternions to Rotation Angles1/1
  Quaternions to Rotation Angles1/1 -> Radians to Degrees13/1
  Radians to Degrees13/1 -> [Simscape_RW_angle]
  PS-Simulink Converter4/1 -> Demux26/1, [Simscape_RW_w]
  PS-Simulink Converter5/1 -> Demux27/1, [Simscape_RW_wd]
  [Torque_ext] -> Simulink-PS Converter1/1
  Demux7/1 -> simscape_angle/1
  Demux7/2 -> simscape_angle/2
  Demux7/3 -> simscape_angle/3
  Quaternions to Rotation Angles2/1 -> Radians to Degrees14/1
  PS-Simulink Converter8/1 -> [Simscape_wd]
  Radians to Degrees14/1 -> [Simscape_angle]
  PS-Simulink Converter7/1 -> [Simscape_w]
  PS-Simulink Converter6/1 -> [Simscape_quat], Quaternions to Rotation Angles2/1
  Constant6/1 -> Rotation Angles to Quaternions1/1
  Quaternion Normalize1/1 -> [RWheel_quat], deriviation of quaternion1/2(q)
  Rotation Angles to Quaternions1/1 -> Integrator3/2
  deriviation of quaternion1/1(q_prime) -> Integrator3/1
  Integrator3/1 -> Quaternion Normalize1/1
  Quaternions to Rotation Angles5/1 -> Radians to Degrees26/1
  Radians to Degrees26/1 -> Demux22/1
  Demux18/3 -> Sum7/2
  Demux17/1 -> Scope8/1
  Sum7/1 -> diff_sim_eq/3
  [Euler_eq_w] -> Demux17/1
  Sum6/1 -> diff_sim_eq/2
  [Simscape_w] -> Demux19/1
  Demux17/2 -> Scope8/2
  [Simscape_wd] -> Demux20/1
  [Simscape_angle] -> Demux21/1
  Sum8/1 -> Sum4/1, diff_sim_eq/1
  Demux20/3 -> Sum7/1
  Demux21/1 -> Sum8/1
  Demux19/3 -> Sum6/1
  [Euler_eq_wd] -> Demux18/1
  Demux17/3 -> Sum6/2, Scope8/3
  Demux22/1 -> Sum8/2
  [Euler_eq_quat] -> Quaternions to Rotation Angles5/1
  Demux5/3 -> Sum1/1
  Demux3/3 -> Sum1/2, Scope6/3
  Demux9/1 -> Sum9/2
  [RWheel_wd] -> Demux4/1
  Demux8/1 -> Sum9/1
  Demux3/2 -> Scope6/2
  Demux6/3 -> Sum2/1
  [Simscape_RW_wd] -> Demux6/1
  Sum9/1 -> Sum3/1, diff_RW_sim_eq/1
  Quaternions to Rotation Angles3/1 -> Radians to Degrees12/1
  Sum2/1 -> diff_RW_sim_eq/3
  [RWheel_w] -> Demux3/1
  [RWheel_quat] -> Quaternions to Rotation Angles3/1
  Demux4/3 -> Sum2/2
  Demux3/1 -> Scope6/1
  [Simscape_RW_w] -> Demux5/1
  Radians to Degrees12/1 -> Demux9/1
  Sum1/1 -> (rad/sec) to RPM5/1
  Demux10/3 -> Simulink-PS Converter/1
  [control_input_Torque] -> Demux10/1
  Constant/1 -> ?
  [Simscape_RW_angle] -> Demux11/1, Demux8/1
  Demux11/1 -> Simscape_RW_angle/1
  Demux11/2 -> Simscape_RW_angle/2
  Demux11/3 -> Simscape_RW_angle/3
  Quaternions to Rotation Angles4/1 -> Radians to Degrees2/1
  [RWheel_quat] -> Quaternions to Rotation Angles4/1
  Radians to Degrees2/1 -> Demux12/1, Eq_Reaction wheel/1
  Demux12/1 -> Euler_RW_angle/1
  Demux12/2 -> Euler_RW_angle/2
  Demux12/3 -> Euler_RW_angle/3
  [RWheel_quat] -> Quaternion Inverse/1
  Quaternion Inverse/1 -> Quaternion Multiplication/2
  Quaternion Multiplication/1 -> Quaternions to Rotation Angles6/1
  [Simscape_RW_quat] -> Quaternion Multiplication/1
  Quaternions to Rotation Angles6/1 -> Radians to Degrees5/1
  Demux13/1 -> Sum3/2, diff_RW_sim_eq_angle/1
  Demux13/2 -> diff_RW_sim_eq_angle/2
  Demux13/3 -> diff_RW_sim_eq_angle/3
  Demux14/2 -> diff_sim_eq_angle/2
  Demux14/3 -> diff_sim_eq_angle/3
  Quaternions to Rotation Angles7/1 -> Radians to Degrees1/1
  [Simscape_quat] -> Quaternion Multiplication1/1
  Quaternion Multiplication1/1 -> Quaternions to Rotation Angles7/1
  Demux14/1 -> diff_sim_eq_angle/1, Sum4/2
  [Euler_eq_quat] -> Quaternion Inverse1/1
  Quaternion Inverse1/1 -> Quaternion Multiplication1/2
  Demux15/2 -> diff_RW_sim_eq_quat/2
  Demux15/3 -> diff_RW_sim_eq_quat/3
  [RWheel_quat] -> Quaternion Inverse2/1
  Demux15/1 -> diff_RW_sim_eq_quat/1
  Quaternion Inverse3/1 -> Quaternion Multiplication3/2
  Demux16/1 -> diff_sim_eq_qaut/1
  Demux16/3 -> diff_sim_eq_qaut/3
  Demux16/2 -> diff_sim_eq_qaut/2
  [Euler_eq_quat] -> Quaternion Inverse3/1
  [Simscape_RW_quat] -> Quaternion Multiplication2/1
  [Simscape_quat] -> Quaternion Multiplication3/1
  Quaternion Multiplication2/1 -> Demux15/1
  Quaternion Multiplication3/1 -> Demux16/1
  Quaternion Inverse2/1 -> Quaternion Multiplication2/2
  Demux16/4 -> diff_sim_eq_qaut/4
  Demux15/4 -> diff_RW_sim_eq_quat/4
  (rad/sec) to RPM/1 -> Simscape/2
  (rad/sec) to RPM1/1 -> Euler_eq/2
  (rad/sec) to RPM2/1 -> Eq_Reaction wheel/2
  (rad/sec) to RPM3/1 -> Simscape_RW/2
  [Simscape_RW_angle] -> Demux23/1, Simscape_RW/1
  [Simscape_RW_wd] -> Simscape_RW/3
  Demux23/1 -> simscape_RW_angle/1
  Demux23/2 -> simscape_RW_angle/2
  [Simscape_RW_w] -> (rad/sec) to RPM3/1
  Demux23/3 -> simscape_RW_angle/3
  Radians to Degrees1/1 -> Demux14/1
  Radians to Degrees5/1 -> Demux13/1
  Sum3/1 -> angle_differ_differ/1
  Sum4/1 -> Sum/1, angle_differ_differ1/1
  [Torque_ext] -> rigid body2/2(t_ext)
  rigid body2/1(omega_prime) -> Add1/2, Add2/1, Integrator4/1
  Constant7/1 -> Degrees to Radians2/1
  Degrees to Radians2/1 -> Integrator4/2
  [Simscape_w] -> Scope/2, Add/2
  Add/1 -> Scope/3
  [Simscape_wd] -> Add1/1
  Add1/1 -> Scope1/1
  PS-Simulink Converter9/1 -> rigid body2/1(Ib), Display/1
  Constant8/1 -> Integrator5/1, Simulink-PS Converter2/3
  Integrator5/1 -> Integrator6/1, Simulink-PS Converter2/2
  Integrator6/1 -> Simulink-PS Converter2/1
  Quaternion Normalize2/1 -> quaternion to Euler angle 1/1(q), deriviation of quaternion2/2(q)
  Demux24/2 -> Scope2/2
  Demux24/3 -> Scope2/3
  Constant9/1 -> Rotation Angles to Quaternions2/1
  Demux24/1 -> Sum5/2, Scope2/1
  Integrator4/1 -> rigid body2/3(omega), (rad/sec) to RPM4/1, deriviation of quaternion2/1(w), Add/1
  quaternion to Euler angle 1/1(angle) -> Radians to Degrees6/1
  Integrator7/1 -> Quaternion Normalize2/1
  deriviation of quaternion2/1(q_prime) -> Integrator7/1
  Radians to Degrees6/1 -> Demux24/1
  Rotation Angles to Quaternions2/1 -> Integrator7/2
  (rad/sec) to RPM4/1 -> Scope/1
  [Simscape_angle] -> Demux25/1
  Demux25/1 -> Sum5/1
  Sum5/1 -> Sum/2, Scope3/1
  Sum/1 -> Scope4/1
  Sum10/1 -> Scope7/1
  Demux26/3 -> Sum10/1
  Sum11/1 -> Scope9/1
  Demux27/3 -> Sum11/1
  Constant3/1 -> Gain/1
  Reshape/1 -> rigid body2/4(omega_rw)
  Reshape1/1 -> Display2/1, Add3/1, rigid body2/5(omega_rw_prime)
  Add2/1 -> Scope11/1
  [Simscape_RW_w] -> rigid body/3(omega_rw)
  [Simscape_RW_wd] -> rigid body/4(omega_rw_prime)
  PS-Simulink Converter10/1 -> [I_rw], Display1/1
  [I_rw] -> rigid body1/1(I_rw)
  Add3/1 -> Scope12/1
  (rad/sec) to RPM5/1 -> diff_RW_sim_eq/2
  Gain/1 -> [Torque_ext]
  Mux/1 -> Reshape/1
  Mux1/1 -> Reshape1/1
  [Revolute_Joint_RW_w] -> Mux/3
  Constant10/1 -> Mux1/2, Mux1/1, Mux/2, Mux/1
  [Revolute_Joint_RW_wd] -> Mux1/3
  connections:
  Sticker2/LConn1 -- Rigid Transform1/RConn1
  PS-Simulink Converter1/LConn1 -- Revolute Joint/RConn3
  Revolute Joint/RConn4 -- PS-Simulink Converter2/LConn1
  Sticker3/LConn1 -- Rigid Transform2/RConn1
  Solver Configuration/RConn1 -- 6-DOF Joint/LConn1 -- World Frame/RConn1 -- Mechanism Configuration/RConn1
  Rigid Transform1/LConn1 -- Rigid Transform3/LConn1 -- Rigid Transform2/LConn1 -- Fly_Wheel/LConn1 -- Inertia Sensor1/LConn1 -- Rigid Transform/LConn1
  Rigid Transform/RConn1 -- Sticker1/LConn1
  PS-Simulink Converter/LConn1 -- Revolute Joint/RConn2
  Base1/LConn1 -- Inertia Sensor/LConn1 -- External Force and Torque/RConn1 -- Revolute Joint/LConn1 -- Transform Sensor1/RConn1
  Sticker4/LConn1 -- Rigid Transform3/RConn1
  Revolute Joint/RConn1 -- Transform Sensor/RConn1 -- Fly_Wheel/RConn1
  6-DOF Joint/RConn1 -- Base1/RConn1
  Transform Sensor/RConn2 -- PS-Simulink Converter3/LConn1
  PS-Simulink Converter4/LConn1 -- Transform Sensor/RConn3
  Transform Sensor/RConn4 -- PS-Simulink Converter5/LConn1
  Simulink-PS Converter1/RConn1 -- External Force and Torque/LConn1
  Transform Sensor1/RConn4 -- PS-Simulink Converter8/LConn1
  Transform Sensor1/RConn2 -- PS-Simulink Converter6/LConn1
  PS-Simulink Converter7/LConn1 -- Transform Sensor1/RConn3
  Simulink-PS Converter/RConn1 -- Revolute Joint/LConn2
  PS-Simulink Converter9/LConn1 -- Inertia Sensor/RConn1
  Simulink-PS Converter2/RConn1 -- Revolute Joint1/LConn2
  Inertia Sensor1/RConn1 -- PS-Simulink Converter10/LConn1
